simulink model "Vehicle_Model_2Track_ABS_ESP_KINOBS_EMPTY"  (R2023a)
settings: Solver=ode2  StartTime=T0  StopTime=Tf  FixedStep=Ts  EnableMultiTasking=on
model workspace (MAT data in the model file):
  aKalman = Simulink.Parameter
  aKalman.DataType = 'auto'
  aKalman.Complexity = 'real'
  aKalman.Dimensions = [0 0]
  slipEnabler = Simulink.Parameter
  slipEnabler.DataType = 'auto'
  slipEnabler.Complexity = 'real'
  slipEnabler.Dimensions = [0 0]
values from neighbouring files (symbols this model uses):
  enable_onlinePlots = 0    [run_simulation.m]
  enable_zoom = 1    [run_simulation.m]
  LLC_sampleTime = LLC.sample_time    [run_simulation.m]
  longCTRparam = longitController()    [run_simulation.m]
  previewPointParams = previewPointControllerParams()    [run_simulation.m]
  road_data_sampled = [scenario_data.path.x_sampled', scenario_data.path.y_sampled']    [run_simulation.m]
  scenario_data = load(strcat('./Scenario/', scenario_name , '.mat'))    [run_simulation.m]
  T0 = scenario_data.times.t0    [run_simulation.m]
  tau_delta = vehicle_data.steering_system.tau_D    [run_simulation.m]
  Tf = scenario_data.times.tf    [run_simulation.m]
  Ts = scenario_data.times.step_size*100    [run_simulation.m]
  vehicle_data = getVehicleDataStruct()    [run_simulation.m]
  X0 = loadInitialConditions(scenario_data.vehicle_control.max_speed/3.6)    [run_simulation.m]
undefined symbols (not defined in the file or in its folder): DiscIntNeverNeededParam, latContr_select
libraries: simulink_extras x20, simulink x9, drivingvehiclecontroller x2
(part 1 of 2)
settings Model: Creator=Edoardo  LastModifiedBy=Alessandro
settings SolverCC: AlgebraicLoopSolver=TrustRegion
settings DataIOCC: LimitDataPoints=on  SaveFormat=Array
settings OptimizationCC: DefaultParameterBehavior=Inlined  ReuseModelBlockBuffer=off  PassReuseOutputArgsAs=Individual arguments  MaxStackSize=64  EfficientTunableParamExpr=on
settings DebuggingCC: ReadBeforeWriteMsg=DisableAll  WriteAfterWriteMsg=DisableAll  WriteAfterReadMsg=DisableAll  MultiTaskDSMMsg=none  ParameterTunabilityLossMsg=error  UnconnectedInputMsg=warning  UnconnectedOutputMsg=warning  UnconnectedLineMsg=warning  PregeneratedLibrarySubsystemCodeDiagnostic=none  SFUnexpectedBacktrackingDiag=warning  SFNoUnconditionalDefaultTransitionDiag=warning  SFExecutionAtInitializationDiag=none  ArithmeticOperatorsInVariantConditions=warning
settings HardwareCC: ProdBitPerInt=16  ProdBitPerPointer=16  ProdBitPerSizeT=16  ProdBitPerPtrDiffT=16  ProdLargestAtomicFloat=None  ProdWordSize=16  ProdHWDeviceType=STMicroelectronics->ST10/Super10
settings ModelReferenceCC: UpdateModelReferenceTargets=IfOutOfDate  EnableRefExpFcnMdlSchedulingChecks=on  PropagateSignalLabelsOutOfModel=off
settings SFSimCC: SFSimEcho=off  SimUseLocalCustomCode=off  MATLABDynamicMemAlloc=off  CustomCodeUndefinedFunction=UseInterfaceOnly
settings RTWCC: Description=Embedded Coder  SystemTargetFile=ert.tlc  TemplateMakefile=ert_default_tmf  GenerateReport=on  RetainRTWFile=on  RTWUseLocalCustomCode=off  Toolchain=GNU Tools for ARM Embedded Processors  BuildConfiguration=Faster Runs  IncludeHyperlinkInReport=on  LaunchReport=on  GenerateTraceInfo=on  GenerateTraceReport=on  GenerateTraceReportSl=on  GenerateTraceReportSf=on  GenerateTraceReportEml=on  DLArmComputeVersion=19.05
settings CodeAppCC: ForceParamTrailComments=on  IgnoreCustomStorageClasses=off  OperatorAnnotations=on  SimulinkDataObjDesc=on  SFDataObjDesc=on  InsertBlockDesc=on
settings ERTTargetCC: CodeReplacementLibrary=ARM Cortex-M (Optimized)  SupportVariableSizeSignals=on  RootIOFormat=Structure reference  ERTCustomFileTemplate=example_file_process.tlc
settings ConfigComp: CovMetricSettings=dw  CovSaveCumulativeToWorkspaceVar=on  CovSaveSingleToWorkspaceVar=on  CovExternalEMLEnable=off

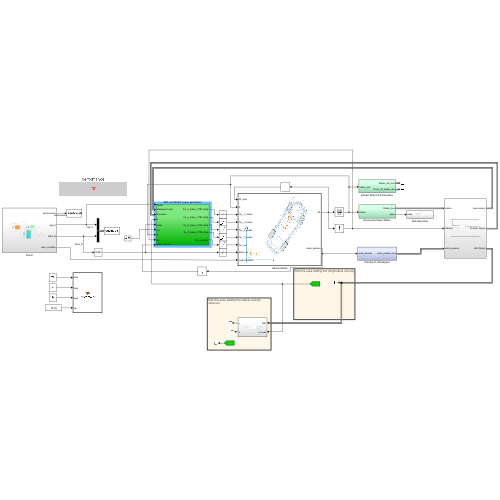
[thumbnail: Simulink's stored preview of the top-level diagram]
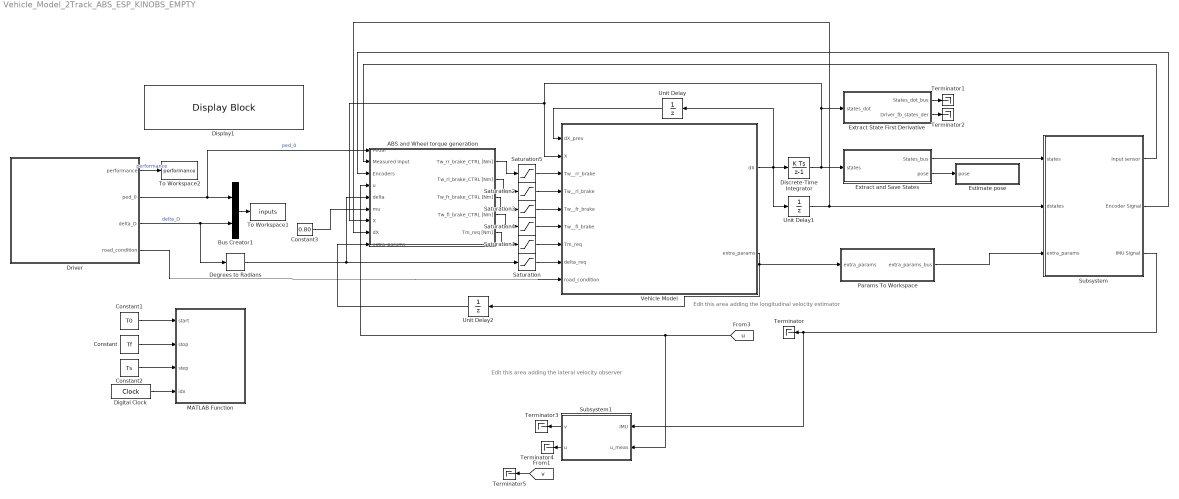
== system Vehicle_Model_2Track_ABS_ESP_KINOBS_EMPTY ==
  note: Edit this area adding the longitudinal velocity estimator
  note: Edit this area adding the lateral velocity
      | observer
  ABS and Wheel torque generation : Subsystem
  Bus Creator1 : BusCreator  Inputs=2
  Constant : Constant  Value=Tf
  Constant1 : Constant  Value=T0
  Constant2 : Constant  Value=Ts
  Constant3 : Constant  Value=0.80
  Degrees to Radians : simulink_extras/Transformations/Degrees to Radians
  Digital Clock : DigitalClock
  Discrete-Time Integrator : DiscreteIntegrator  gainval=1  InitialCondition=X0  SampleTime=-1  ICPrevOutput=DiscIntNeverNeededParam  ICPrevScaledInput=DiscIntNeverNeededParam
  Display1 : DisplayBlock  Format=Integer  Transparency=1  Layout=Fill available space
  Driver : Subsystem
  Estimate pose : Subsystem
  Extract State First Derivative : Subsystem
  Extract and Save States : Subsystem
  MATLAB Function : MATLAB Function  TreatAsAtomicUnit=on
  Params To Workspace : Subsystem
  Saturation : Saturate  UpperLimit=7  LowerLimit=-7
  Saturation1 : Saturate  UpperLimit=vehicle_data.motor.maxTorque  LowerLimit=0
  Saturation{2..5} (4 alike) : Saturate  UpperLimit=0  LowerLimit=-vehicle_data.braking.totBrakeTorque
  Subsystem : Subsystem
  Subsystem1 : Subsystem
  Terminator{,1..5} (6 alike) : Terminator
  To Workspace1 : ToWorkspace  VariableName=inputs  SaveFormat=Timeseries  SampleTime=-1
  To Workspace2 : ToWorkspace  VariableName=performance  SaveFormat=Timeseries  SampleTime=-1
  Unit Delay : UnitDelay  InitialCondition=zeros(size(X0))  SampleTime=-1  HasFrameUpgradeWarning=on
  Unit Delay1 : UnitDelay  InitialCondition=zeros(size(X0))  SampleTime=-1  HasFrameUpgradeWarning=on
  Unit Delay2 : UnitDelay  InitialCondition=zeros(size(X0))  SampleTime=-1  HasFrameUpgradeWarning=on
  Vehicle Model : MATLAB Function  TreatAsAtomicUnit=on
  wires:
  ABS and Wheel torque generation/1(Tw_rr_brake_CTRL [Nm]) -> Saturation5/1
  Subsystem/1(Input sensor) -> ABS and Wheel torque generation/2(Measured Input)
  Degrees to Radians/1 -> ABS and Wheel torque generation/5(delta), Saturation/1
  Bus Creator1/1 -> To Workspace1/1
  Extract and Save States/1(States_bus) -> Subsystem/1(states)
  ABS and Wheel torque generation/3(Tw_fr_brake_CTRL [Nm]) -> Saturation3/1
  Vehicle Model/1(dX) -> Unit Delay1/1, Unit Delay/1, Discrete-Time Integrator/1
  Extract State First Derivative/2(Driver_fb_states_der) -> Terminator2/1
  Subsystem/2(Encoder Signal) -> ABS and Wheel torque generation/3(Encoders)
  Unit Delay/1 -> Vehicle Model/1(dX_prev)
  Extract State First Derivative/1(States_dot_bus) -> Terminator1/1
  Driver/3(delta_D) -> Degrees to Radians/1, Bus Creator1/2  "delta_D"
  Vehicle Model/2(extra_params) -> Unit Delay2/1, Params To Workspace/1(extra_params)
  ABS and Wheel torque generation/2(Tw_rl_brake_CTRL [Nm]) -> Saturation2/1
  ABS and Wheel torque generation/5(Tm_req [Nm]) -> Saturation1/1
  Driver/2(ped_0) -> ABS and Wheel torque generation/1(Pedal), Bus Creator1/1  "ped_0"
  ABS and Wheel torque generation/4(Tw_fl_brake_CTRL [Nm]) -> Saturation4/1
  Params To Workspace/1(extra_params_bus) -> Subsystem/3(extra_params)
  Constant/1 -> MATLAB Function/2(stop)
  Constant1/1 -> MATLAB Function/1(start)
  Digital Clock/1 -> MATLAB Function/4(idx)
  Constant2/1 -> MATLAB Function/3(step)
  Extract and Save States/2(pose) -> Estimate pose/1(pose)
  [u] -> Subsystem1/2(u_meas), ABS and Wheel torque generation/4(u)
  Saturation/1 -> Vehicle Model/8(delta_req)
  Driver/4(road_condition) -> Vehicle Model/9(road_condition)
  Subsystem/3(IMU Signal) -> Subsystem1/1(IMU), Terminator/1
  Saturation1/1 -> Vehicle Model/7(Tm_req)
  Saturation4/1 -> Vehicle Model/6(Tw__fl_brake)
  Saturation3/1 -> Vehicle Model/5(Tw__fr_brake)
  Saturation2/1 -> Vehicle Model/4(Tw__rl_brake)
  Saturation5/1 -> Vehicle Model/3(Tw__rr_brake)
  Driver/1(performance) -> To Workspace2/1  "performance"
  Unit Delay1/1 -> ABS and Wheel torque generation/8(dX), Subsystem/2(dstates)
  [v] -> Terminator5/1
  Constant3/1 -> ABS and Wheel torque generation/6(mu)
  Subsystem1/1(v) -> Terminator3/1
  Subsystem1/2(u) -> Terminator4/1
  Unit Delay2/1 -> ABS and Wheel torque generation/9(extra_params)
  Discrete-Time Integrator/1 -> Extract and Save States/1(states), Extract State First Derivative/1(states_dot), ABS and Wheel torque generation/7(X), Vehicle Model/2(X)

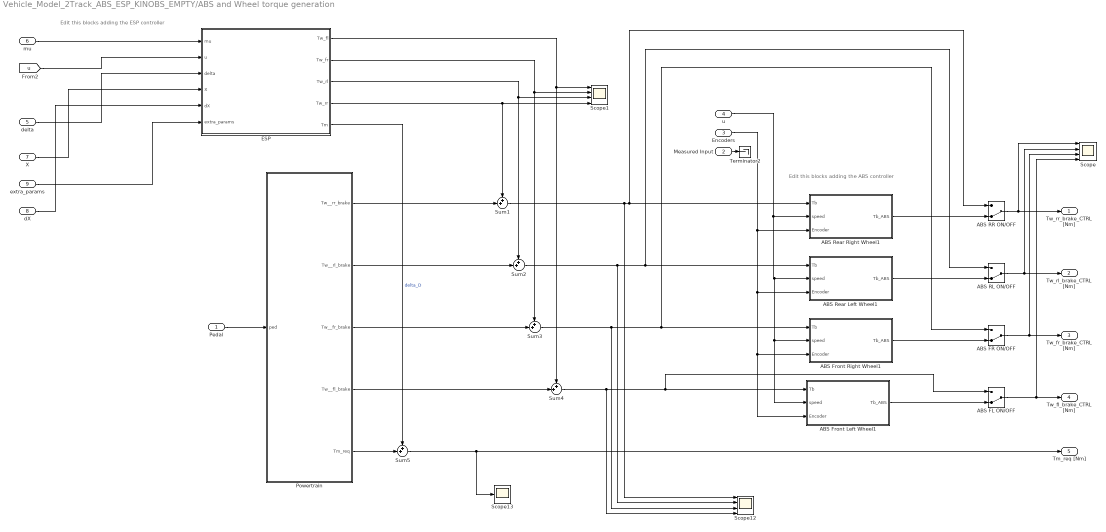
== system Vehicle_Model_2Track_ABS_ESP_KINOBS_EMPTY/ABS and Wheel torque generation ==
  note: Edit this blocks adding the ESP controller
  note: Edit this blocks adding the ABS controller
  Pedal : Inport
  Measured Input : Inport  Port=2
  Encoders : Inport  Port=3
  u : Inport  Port=4
  delta : Inport  Port=5
  mu : Inport  Port=6
  X : Inport  Port=7
  dX : Inport  Port=8
  extra_params : Inport  Port=9
  ABS FL ON/OFF : ManualSwitch  CurrentSetting=0
  ABS FR ON/OFF : ManualSwitch  CurrentSetting=0
  ABS Front Left Wheel1 : Subsystem
  ABS Front Right Wheel1 : Subsystem
  ABS RL ON/OFF : ManualSwitch  CurrentSetting=0
  ABS RR ON/OFF : ManualSwitch  CurrentSetting=0
  ABS Rear Left Wheel1 : Subsystem
  ABS Rear Right Wheel1 : Subsystem
  ESP : Subsystem
  Powertrain : MATLAB Function  TreatAsAtomicUnit=on
  Scope : Scope  NumInputPorts=4
  Scope1 : Scope  NumInputPorts=4
  Scope12 : Scope  NumInputPorts=4
  Scope13 : Scope
  Sum{1..5} (5 alike) : Sum  Inputs=++|
  Terminator2 : Terminator
  Tw_rr_brake_CTRL [Nm] : Outport  VectorParamsAs1DForOutWhenUnconnected=off
  Tw_rl_brake_CTRL [Nm] : Outport  Port=2  VectorParamsAs1DForOutWhenUnconnected=off
  Tw_fr_brake_CTRL [Nm] : Outport  Port=3  VectorParamsAs1DForOutWhenUnconnected=off
  Tw_fl_brake_CTRL [Nm] : Outport  Port=4  VectorParamsAs1DForOutWhenUnconnected=off
  Tm_req [Nm] : Outport  Port=5  VectorParamsAs1DForOutWhenUnconnected=off
  wires:
  Sum3/1 -> Scope12/3, ABS Front Right Wheel1/1(Tb), ABS FR ON/OFF/1
  ABS FL ON/OFF/1 -> Tw_fl_brake_CTRL [Nm]/1, Scope/4
  Sum5/1 -> Scope13/1, Tm_req [Nm]/1
  ABS FR ON/OFF/1 -> Tw_fr_brake_CTRL [Nm]/1, Scope/3
  u/1 -> ABS Rear Right Wheel1/2(speed), ABS Rear Left Wheel1/2(speed), ABS Front Right Wheel1/2(speed), ABS Front Left Wheel1/2(speed)
  ABS RL ON/OFF/1 -> Tw_rl_brake_CTRL [Nm]/1, Scope/2
  Sum2/1 -> Scope12/2, ABS Rear Left Wheel1/1(Tb), ABS RL ON/OFF/1
  Pedal/1 -> Powertrain/1(ped)
  ABS RR ON/OFF/1 -> Scope/1, Tw_rr_brake_CTRL [Nm]/1
  Encoders/1 -> ABS Rear Right Wheel1/3(Encoder), ABS Rear Left Wheel1/3(Encoder), ABS Front Right Wheel1/3(Encoder), ABS Front Left Wheel1/3(Encoder)
  Measured Input/1 -> Terminator2/1
  Sum4/1 -> ABS FL ON/OFF/1, ABS Front Left Wheel1/1(Tb), Scope12/4
  ABS Front Left Wheel1/1(Tb_ABS) -> ABS FL ON/OFF/2
  Sum1/1 -> Scope12/1, ABS Rear Right Wheel1/1(Tb), ABS RR ON/OFF/1
  Powertrain/1(Tw__rr_brake) -> Sum1/2
  Powertrain/2(Tw__rl_brake) -> Sum2/2
  Powertrain/3(Tw__fr_brake) -> Sum3/2
  Powertrain/4(Tw__fl_brake) -> Sum4/2
  Powertrain/5(Tm_req) -> Sum5/2
  ESP/5(Tm) -> Sum5/1  "delta_D"
  ESP/1(Tw_fl) -> Sum4/1, Scope1/1
  ESP/3(Tw_rl) -> Sum2/1, Scope1/3
  ESP/2(Tw_fr) -> Sum3/1, Scope1/2
  ESP/4(Tw_rr) -> Sum1/1, Scope1/4
  mu/1 -> ESP/1(mu)
  [u] -> ESP/2(u)
  delta/1 -> ESP/3(delta)
  ABS Front Right Wheel1/1(Tb_ABS) -> ABS FR ON/OFF/2
  ABS Rear Left Wheel1/1(Tb_ABS) -> ABS RL ON/OFF/2
  ABS Rear Right Wheel1/1(Tb_ABS) -> ABS RR ON/OFF/2
  X/1 -> ESP/4(X)
  dX/1 -> ESP/5(dX)
  extra_params/1 -> ESP/6(extra_params)

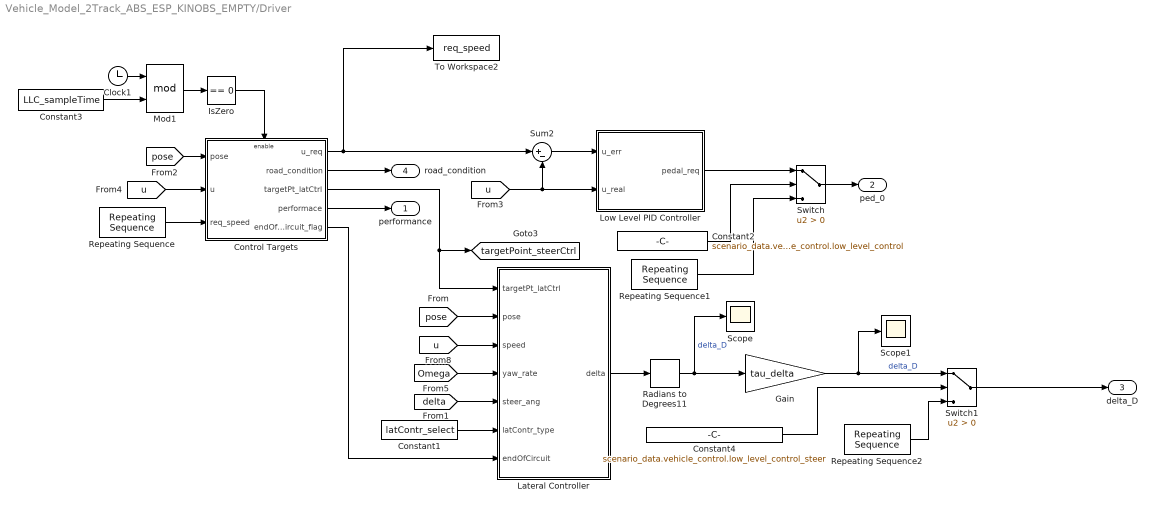
== system Vehicle_Model_2Track_ABS_ESP_KINOBS_EMPTY/Driver ==
  Clock1 : Clock
  Constant1 : Constant  Value=latContr_select
  Constant2 : Constant  Value=scenario_data.vehicle_control.low_level_control
  Constant3 : Constant  Value=LLC_sampleTime
  Constant4 : Constant  Value=scenario_data.vehicle_control.low_level_control_steer
  Control Targets : Subsystem
  Gain : Gain  Gain=tau_delta
  IsZero : simulink/Logic and Bit Operations/Compare To Zero  relop===  OutDataTypeStr=boolean
  Lateral Controller : Subsystem
  Low Level PID Controller : Subsystem
  Mod1 : Math  Operator=mod  SignedPower=on
  Radians to Degrees11 : simulink_extras/Transformations/Radians to Degrees
  Repeating Sequence : simulink/Sources/Repeating Sequence  rep_seq_t=scenario_data.vehicle_control.time_manoeuvre  rep_seq_y=scenario_data.vehicle_control.req_speed
  Repeating Sequence1 : simulink/Sources/Repeating Sequence  rep_seq_t=scenario_data.vehicle_control.time_pedal  rep_seq_y=scenario_data.vehicle_control.req_pedal
  Repeating Sequence2 : simulink/Sources/Repeating Sequence  rep_seq_t=scenario_data.vehicle_control.time_delta  rep_seq_y=scenario_data.vehicle_control.req_delta
  Scope : Scope
  Scope1 : Scope
  Sum2 : Sum  Inputs=|+-
  Switch : Switch  Criteria=u2 > Threshold  SaturateOnIntegerOverflow=off  InputSameDT=off
  Switch1 : Switch  Criteria=u2 > Threshold  SaturateOnIntegerOverflow=off  InputSameDT=off
  To Workspace2 : ToWorkspace  VariableName=req_speed  SaveFormat=Timeseries  SampleTime=-1
  performance : Outport
  ped_0 : Outport  Port=2  PortDimensions=1
  delta_D : Outport  Port=3  PortDimensions=1
  road_condition : Outport  Port=4
  tag scope: targetPoint_steerCtrl=global
  wires:
  Constant1/1 -> Lateral Controller/6(latContr_type)
  [pose] -> Lateral Controller/2(pose)
  [pose] -> Control Targets/1(pose)
  IsZero/1 -> Control Targets/Enable
  [u] -> Lateral Controller/3(speed)
  [u] -> Sum2/2, Low Level PID Controller/2(u_real)
  Clock1/1 -> Mod1/1
  Control Targets/1(u_req) -> Sum2/1, To Workspace2/1
  [Omega] -> Lateral Controller/4(yaw_rate)
  Sum2/1 -> Low Level PID Controller/1(u_err)
  Constant3/1 -> Mod1/2
  Mod1/1 -> IsZero/1
  Control Targets/3(targetPt_latCtrl) -> Lateral Controller/1(targetPt_latCtrl), [targetPoint_steerCtrl]
  [delta] -> Lateral Controller/5(steer_ang)
  Lateral Controller/1(delta) -> Radians to Degrees11/1
  Control Targets/5(endOfCircuit_flag) -> Lateral Controller/7(endOfCircuit)
  Gain/1 -> Switch1/1, Scope1/1  "delta_D"
  Repeating Sequence/1 -> Control Targets/3(req_speed)
  Switch/1 -> ped_0/1
  Repeating Sequence1/1 -> Switch/3
  Low Level PID Controller/1(pedal_req) -> Switch/1
  Radians to Degrees11/1 -> Gain/1, Scope/1  "delta_D"
  Control Targets/2(road_condition) -> road_condition/1
  Constant2/1 -> Switch/2
  Constant4/1 -> Switch1/2
  Repeating Sequence2/1 -> Switch1/3
  Switch1/1 -> delta_D/1
  [u] -> Control Targets/2(u)
  Control Targets/4(performace) -> performance/1

== system Vehicle_Model_2Track_ABS_ESP_KINOBS_EMPTY/Estimate pose ==
  pose : Inport
  Constant3 : Constant  Value=enable_onlinePlots
  Online Trajectory Plots : Subsystem
      mask Display: image('example_path.png'); % Use "Edit Image" on toolstrip to change.
  To Workspace4 : ToWorkspace  VariableName=vehicle_pose  SampleTime=-1
      settings: Save2DSignal=2-D array (concatenate along first dimension)
  wires:
  [targetPoint_steerCtrl] -> Online Trajectory Plots/1(targetPoint_steerCtrl)
  Constant3/1 -> Online Trajectory Plots/Enable
  pose/1 -> To Workspace4/1, Online Trajectory Plots/2(pose)

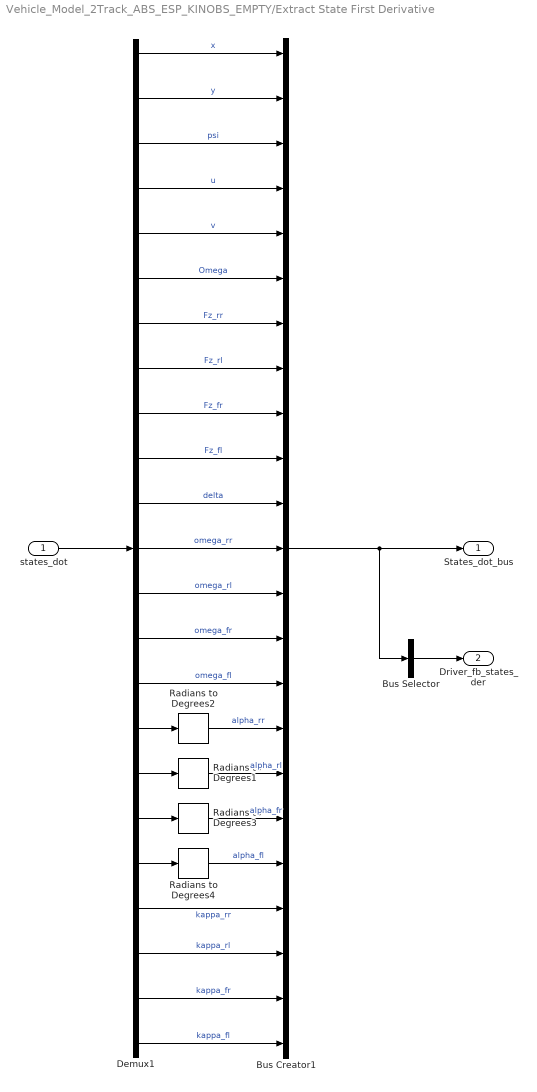
== system Vehicle_Model_2Track_ABS_ESP_KINOBS_EMPTY/Extract State First Derivative ==
  states_dot : Inport
  Bus Creator1 : BusCreator  Inputs=23
  Bus Selector : BusSelector  OutputSignals=Omega,x,y,u  OutputAsBus=on
  Demux1 : Demux  Outputs=23
  Radians to Degrees{1..4} (4 alike) : simulink_extras/Transformations/Radians to Degrees
  States_dot_bus : Outport
  Driver_fb_states_der : Outport  Port=2
  wires:
  Demux1/13 -> Bus Creator1/13  "omega_rl"
  Demux1/8 -> Bus Creator1/8  "Fz_rl"
  Demux1/23 -> Bus Creator1/23  "kappa_fl"
  Demux1/19 -> Radians to Degrees4/1
  states_dot/1 -> Demux1/1
  Demux1/14 -> Bus Creator1/14  "omega_fr"
  Demux1/7 -> Bus Creator1/7  "Fz_rr"
  Demux1/15 -> Bus Creator1/15  "omega_fl"
  Demux1/3 -> Bus Creator1/3  "psi"
  Demux1/22 -> Bus Creator1/22  "kappa_fr"
  Demux1/4 -> Bus Creator1/4  "u"
  Demux1/6 -> Bus Creator1/6  "Omega"
  Demux1/11 -> Bus Creator1/11  "delta"
  Demux1/5 -> Bus Creator1/5  "v"
  Demux1/9 -> Bus Creator1/9  "Fz_fr"
  Demux1/21 -> Bus Creator1/21  "kappa_rl"
  Demux1/12 -> Bus Creator1/12  "omega_rr"
  Demux1/17 -> Radians to Degrees1/1
  Demux1/2 -> Bus Creator1/2  "y"
  Demux1/20 -> Bus Creator1/20  "kappa_rr"
  Demux1/10 -> Bus Creator1/10  "Fz_fl"
  Demux1/18 -> Radians to Degrees3/1
  Demux1/1 -> Bus Creator1/1  "x"
  Demux1/16 -> Radians to Degrees2/1
  Bus Creator1/1 -> Bus Selector/1, States_dot_bus/1
  Radians to Degrees2/1 -> Bus Creator1/16  "alpha_rr"
  Radians to Degrees1/1 -> Bus Creator1/17  "alpha_rl"
  Radians to Degrees3/1 -> Bus Creator1/18  "alpha_fr"
  Radians to Degrees4/1 -> Bus Creator1/19  "alpha_fl"
  Bus Selector/1 -> Driver_fb_states_der/1

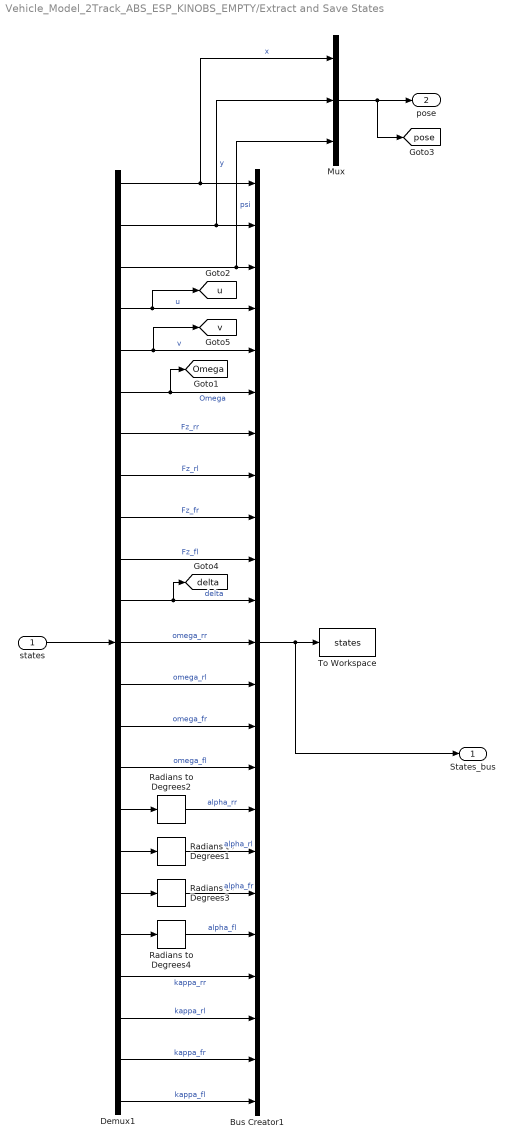
== system Vehicle_Model_2Track_ABS_ESP_KINOBS_EMPTY/Extract and Save States ==
  states : Inport
  Bus Creator1 : BusCreator  Inputs=23
  Demux1 : Demux  Outputs=23
  Mux : Mux  Inputs=3
  Radians to Degrees{1..4} (4 alike) : simulink_extras/Transformations/Radians to Degrees
  To Workspace : ToWorkspace  VariableName=states  SaveFormat=Timeseries  SampleTime=-1
  States_bus : Outport
  pose : Outport  Port=2
  tag scope: Omega=global, delta=global, pose=global, u=global, v=global
  wires:
  Demux1/13 -> Bus Creator1/13  "omega_rl"
  Demux1/8 -> Bus Creator1/8  "Fz_rl"
  Demux1/23 -> Bus Creator1/23  "kappa_fl"
  Demux1/19 -> Radians to Degrees4/1
  states/1 -> Demux1/1
  Demux1/14 -> Bus Creator1/14  "omega_fr"
  Demux1/7 -> Bus Creator1/7  "Fz_rr"
  Demux1/15 -> Bus Creator1/15  "omega_fl"
  Demux1/22 -> Bus Creator1/22  "kappa_fr"
  Demux1/6 -> [Omega], Bus Creator1/6  "Omega"
  Demux1/11 -> [delta], Bus Creator1/11  "delta"
  Demux1/5 -> [v], Bus Creator1/5  "v"
  Demux1/9 -> Bus Creator1/9  "Fz_fr"
  Demux1/21 -> Bus Creator1/21  "kappa_rl"
  Demux1/12 -> Bus Creator1/12  "omega_rr"
  Demux1/17 -> Radians to Degrees1/1
  Demux1/20 -> Bus Creator1/20  "kappa_rr"
  Demux1/10 -> Bus Creator1/10  "Fz_fl"
  Demux1/18 -> Radians to Degrees3/1
  Demux1/16 -> Radians to Degrees2/1
  Bus Creator1/1 -> States_bus/1, To Workspace/1
  Radians to Degrees2/1 -> Bus Creator1/16  "alpha_rr"
  Radians to Degrees1/1 -> Bus Creator1/17  "alpha_rl"
  Radians to Degrees3/1 -> Bus Creator1/18  "alpha_fr"
  Radians to Degrees4/1 -> Bus Creator1/19  "alpha_fl"
  Demux1/1 -> Mux/1, Bus Creator1/1  "x"
  Demux1/3 -> Mux/3, Bus Creator1/3  "psi"
  Demux1/4 -> [u], Bus Creator1/4  "u"
  Demux1/2 -> Bus Creator1/2, Mux/2  "y"
  Mux/1 -> [pose], pose/1

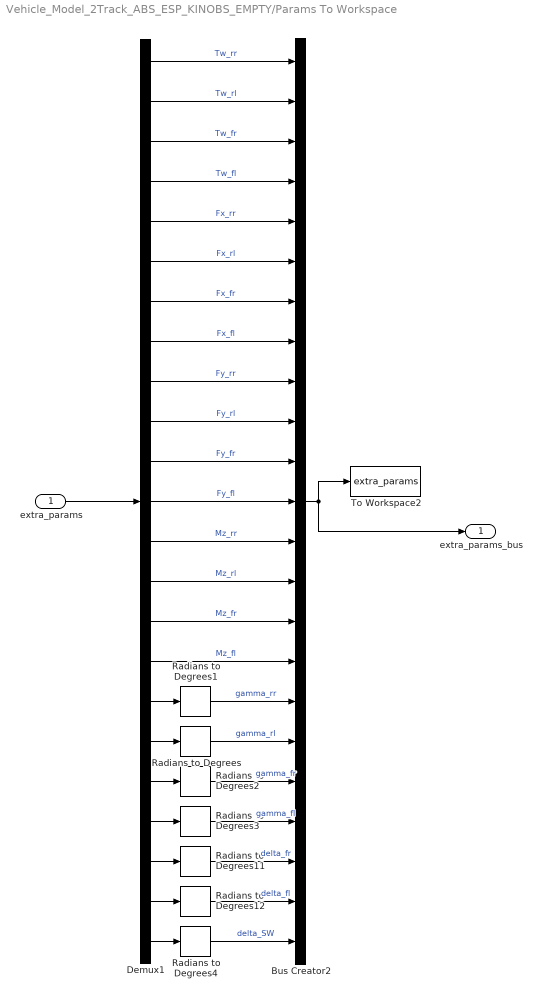
== system Vehicle_Model_2Track_ABS_ESP_KINOBS_EMPTY/Params To Workspace ==
  extra_params : Inport
  Bus Creator2 : BusCreator  Inputs=23
  Demux1 : Demux  Outputs=23
  Radians to Degrees{,1..4,11..12} (7 alike) : simulink_extras/Transformations/Radians to Degrees
  To Workspace2 : ToWorkspace  VariableName=extra_params  SaveFormat=Timeseries  SampleTime=-1
  extra_params_bus : Outport
  wires:
  Demux1/17 -> Radians to Degrees1/1
  Demux1/3 -> Bus Creator2/3  "Tw_fr"
  Radians to Degrees3/1 -> Bus Creator2/20  "gamma_fl"
  Demux1/16 -> Bus Creator2/16  "Mz_fl"
  Radians to Degrees1/1 -> Bus Creator2/17  "gamma_rr"
  Radians to Degrees11/1 -> Bus Creator2/21  "delta_fr"
  Demux1/14 -> Bus Creator2/14  "Mz_rl"
  Demux1/4 -> Bus Creator2/4  "Tw_fl"
  Demux1/6 -> Bus Creator2/6  "Fx_rl"
  Demux1/8 -> Bus Creator2/8  "Fx_fl"
  Demux1/13 -> Bus Creator2/13  "Mz_rr"
  Demux1/7 -> Bus Creator2/7  "Fx_fr"
  Demux1/5 -> Bus Creator2/5  "Fx_rr"
  Demux1/9 -> Bus Creator2/9  "Fy_rr"
  Demux1/11 -> Bus Creator2/11  "Fy_fr"
  Demux1/15 -> Bus Creator2/15  "Mz_fr"
  Demux1/10 -> Bus Creator2/10  "Fy_rl"
  Radians to Degrees12/1 -> Bus Creator2/22  "delta_fl"
  Radians to Degrees2/1 -> Bus Creator2/19  "gamma_fr"
  extra_params/1 -> Demux1/1
  Demux1/12 -> Bus Creator2/12  "Fy_fl"
  Bus Creator2/1 -> To Workspace2/1, extra_params_bus/1
  Demux1/1 -> Bus Creator2/1  "Tw_rr"
  Demux1/2 -> Bus Creator2/2  "Tw_rl"
  Radians to Degrees/1 -> Bus Creator2/18  "gamma_rl"
  Demux1/18 -> Radians to Degrees/1
  Demux1/19 -> Radians to Degrees2/1
  Demux1/20 -> Radians to Degrees3/1
  Demux1/21 -> Radians to Degrees11/1
  Demux1/22 -> Radians to Degrees12/1
  Demux1/23 -> Radians to Degrees4/1
  Radians to Degrees4/1 -> Bus Creator2/23  "delta_SW"

== system Vehicle_Model_2Track_ABS_ESP_KINOBS_EMPTY/Subsystem ==
  states : Inport
  dstates : Inport  Port=2
  extra_params : Inport  Port=3
  Bus Selector : BusSelector  OutputSignals=omega_rr,omega_rl,omega_fr,omega_fl  OutputAsBus=on
  Bus Selector1 : BusSelector  OutputSignals=delta_SW,Tw_rr,Tw_rl,Tw_fr,Tw_fl  OutputAsBus=on
  IMU1 : Subsystem
  Input sensor : Outport  VectorParamsAs1DForOutWhenUnconnected=off
  Encoder Signal : Outport  Port=2  VectorParamsAs1DForOutWhenUnconnected=off
  IMU Signal : Outport  Port=3  VectorParamsAs1DForOutWhenUnconnected=off
  wires:
  states/1 -> IMU1/1(states), Bus Selector/1
  Bus Selector/1 -> Encoder Signal/1
  IMU1/1(IMU) -> IMU Signal/1
  extra_params/1 -> Bus Selector1/1
  Bus Selector1/1 -> Input sensor/1
  dstates/1 -> IMU1/2(dstates)

== system Vehicle_Model_2Track_ABS_ESP_KINOBS_EMPTY/Subsystem1 ==
  IMU : Inport
  u_meas : Inport  Port=2
  Bus Selector : BusSelector  OutputSignals=a_x,a_y,Omega
  Demux : Demux  Outputs=2
  Discrete-Time Integrator : DiscreteIntegrator  InitialCondition=[0 ; 0]  SampleTime=-1  ICPrevOutput=DiscIntNeverNeededParam  ICPrevScaledInput=DiscIntNeverNeededParam
  MATLAB Function : MATLAB Function  TreatAsAtomicUnit=on
  gamma : Constant
  v : Outport
  u : Outport  Port=2
  wires:
  IMU/1 -> Bus Selector/1
  Bus Selector/3 -> MATLAB Function/4(omega)  "<Omega>"
  Bus Selector/2 -> MATLAB Function/3(ay)  "<a_y>"
  Bus Selector/1 -> MATLAB Function/2(ax)  "<a_x>"
  MATLAB Function/1(X_dot) -> Discrete-Time Integrator/1
  Discrete-Time Integrator/1 -> MATLAB Function/1(X), Demux/1
  Demux/1 -> v/1
  Demux/2 -> u/1
  gamma/1 -> MATLAB Function/5(gamma)
  u_meas/1 -> MATLAB Function/6(u_meas)

== system Vehicle_Model_2Track_ABS_ESP_KINOBS_EMPTY/ABS and Wheel torque generation/ABS Front Left Wheel1 ==
  Tb : Inport
  speed : Inport  Port=2
  Encoder : Inport  Port=3
  Terminator : Terminator
  Terminator1 : Terminator
  To Workspace3 : ToWorkspace  VariableName=TwrflCtrl  SaveFormat=Timeseries  SampleTime=-1
  Tb_ABS : Outport  VectorParamsAs1DForOutWhenUnconnected=off
  wires:
  Encoder/1 -> Terminator/1
  Tb/1 -> To Workspace3/1, Tb_ABS/1
  speed/1 -> Terminator1/1

== system Vehicle_Model_2Track_ABS_ESP_KINOBS_EMPTY/ABS and Wheel torque generation/ABS Front Right Wheel1 ==
  Tb : Inport
  speed : Inport  Port=2
  Encoder : Inport  Port=3
  Terminator : Terminator
  Terminator1 : Terminator
  To Workspace3 : ToWorkspace  VariableName=TwfrCtrl  SaveFormat=Timeseries  SampleTime=-1
  Tb_ABS : Outport  VectorParamsAs1DForOutWhenUnconnected=off
  wires:
  Encoder/1 -> Terminator1/1
  Tb/1 -> Tb_ABS/1, To Workspace3/1
  speed/1 -> Terminator/1

== system Vehicle_Model_2Track_ABS_ESP_KINOBS_EMPTY/ABS and Wheel torque generation/ABS Rear Left Wheel1 ==
  Tb : Inport
  speed : Inport  Port=2
  Encoder : Inport  Port=3
  Terminator : Terminator
  Terminator1 : Terminator
  To Workspace3 : ToWorkspace  VariableName=TwrlCtrl  SaveFormat=Timeseries  SampleTime=-1
  Tb_ABS : Outport  VectorParamsAs1DForOutWhenUnconnected=off
  wires:
  Encoder/1 -> Terminator1/1
  Tb/1 -> To Workspace3/1, Tb_ABS/1
  speed/1 -> Terminator/1

== system Vehicle_Model_2Track_ABS_ESP_KINOBS_EMPTY/ABS and Wheel torque generation/ABS Rear Right Wheel1 ==
  Tb : Inport
  speed : Inport  Port=2
  Encoder : Inport  Port=3
  Terminator : Terminator
  Terminator1 : Terminator
  To Workspace3 : ToWorkspace  VariableName=TwrrCtrl  SaveFormat=Timeseries  SampleTime=-1
  Tb_ABS : Outport  VectorParamsAs1DForOutWhenUnconnected=off
  wires:
  Encoder/1 -> Terminator1/1
  Tb/1 -> To Workspace3/1, Tb_ABS/1
  speed/1 -> Terminator/1

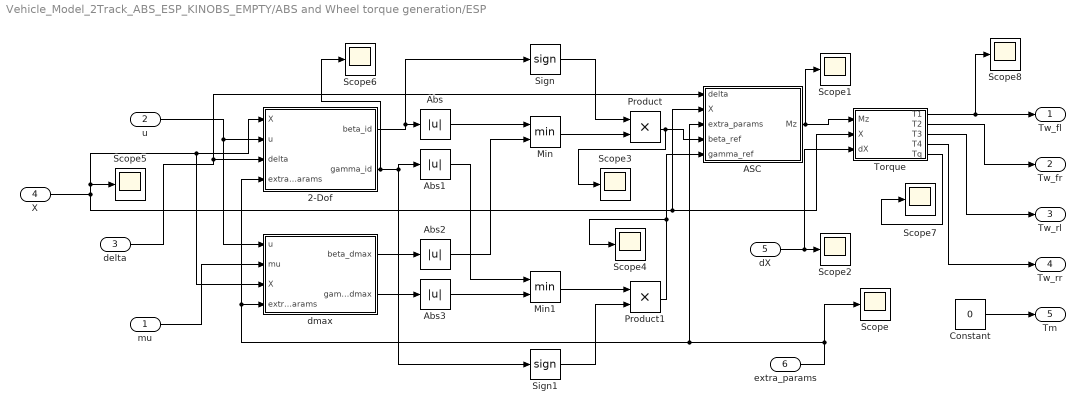
== system Vehicle_Model_2Track_ABS_ESP_KINOBS_EMPTY/ABS and Wheel torque generation/ESP ==
  mu : Inport
  u : Inport  Port=2
  delta : Inport  Port=3
  X : Inport  Port=4
  dX : Inport  Port=5
  extra_params : Inport  Port=6
  2-Dof : MATLAB Function  TreatAsAtomicUnit=on
  ASC : MATLAB Function  TreatAsAtomicUnit=on
  Abs{,1..3} (4 alike) : Abs  SaturateOnIntegerOverflow=off
  Constant : Constant  Value=0
  Min : MinMax  Inputs=2
  Min1 : MinMax  Inputs=2
  Product : Product
  Product1 : Product
  Scope{,1..8} (9 alike) : Scope
  Sign : Signum
  Sign1 : Signum
  Torque : MATLAB Function  TreatAsAtomicUnit=on
  dmax : MATLAB Function  TreatAsAtomicUnit=on
  Tw_fl : Outport
  Tw_fr : Outport  Port=2
  Tw_rl : Outport  Port=3
  Tw_rr : Outport  Port=4
  Tm : Outport  Port=5
  wires:
  mu/1 -> dmax/2(mu)
  dmax/1(beta_dmax) -> Abs2/1
  dmax/2(gamma_dmax) -> Abs3/1
  Abs/1 -> Min/1
  Abs2/1 -> Min/2
  Abs1/1 -> Min1/1
  Abs3/1 -> Min1/2
  Sign/1 -> Product/1
  Min/1 -> Product/2
  Min1/1 -> Product1/1
  Sign1/1 -> Product1/2
  X/1 -> Torque/2(X), ASC/2(X), 2-Dof/1(X), dmax/3(X), Scope5/1
  ASC/1(Mz) -> Scope1/1, Torque/1(Mz)
  dX/1 -> Scope2/1, Torque/3(dX)
  Product/1 -> Scope3/1, ASC/4(beta_ref)
  Product1/1 -> Scope4/1, ASC/5(gamma_ref)
  Constant/1 -> Tm/1
  extra_params/1 -> Scope/1, ASC/3(extra_params), 2-Dof/4(extra_params), dmax/4(extra_params)
  2-Dof/1(beta_id) -> Sign/1, Abs/1
  2-Dof/2(gamma_id) -> Scope6/1, Abs1/1, Sign1/1
  u/1 -> 2-Dof/2(u), dmax/1(u)
  Torque/4(T4) -> Tw_rr/1
  Torque/1(T1) -> Scope8/1, Tw_fl/1
  Torque/3(T3) -> Tw_rl/1
  Torque/2(T2) -> Tw_fr/1
  delta/1 -> 2-Dof/3(delta), ASC/1(delta)
  Torque/5(Tq) -> Scope7/1

== system Vehicle_Model_2Track_ABS_ESP_KINOBS_EMPTY/Driver/Control Targets ==
  pose : Inport
  u : Inport  Port=2
  req_speed : Inport  Port=3
  Enable : EnablePort
  MATLAB System : MATLABSystem  System=setControlTargets  lateralController_type=latContr_select  purePursuit_lookAhead=purePursuitParams.lookAhead  clothoidBased_lookAhead=clothoidBasedParams.lookAhead  previewPoint_lookAhead=previewPointParams.lookAhead  refRoute_points=road_data  road_condition=road_condition  Lf=vehicle_data.vehicle.Lf  SimulateUsing=Interpreted execution
      mask Type: setControlTargets
      mask Display:
      | disp('setControlTargets');
      | port_label('input',1,'vehPose');
      | port_label('input',2,'u');
      | port_label('input',3,'req_speed');
      | port_label('output',1,'targetPoint_latControl');
      | port_label('output',2,'speed_req');
      | port_label('output',3,'road_condition');
      | port_label('output',4,'performance');
      | port_label('output',5,'endOfCircuit');
  u_req : Outport  VectorParamsAs1DForOutWhenUnconnected=off
  road_condition : Outport  Port=2
  targetPt_latCtrl : Outport  Port=3  VectorParamsAs1DForOutWhenUnconnected=off
  performace : Outport  Port=4  VectorParamsAs1DForOutWhenUnconnected=off
  endOfCircuit_flag : Outport  Port=5  VectorParamsAs1DForOutWhenUnconnected=off
  wires:
  pose/1 -> MATLAB System/1
  MATLAB System/2 -> u_req/1
  MATLAB System/1 -> targetPt_latCtrl/1
  MATLAB System/4 -> performace/1
  req_speed/1 -> MATLAB System/3
  MATLAB System/3 -> road_condition/1
  u/1 -> MATLAB System/2
  MATLAB System/5 -> endOfCircuit_flag/1

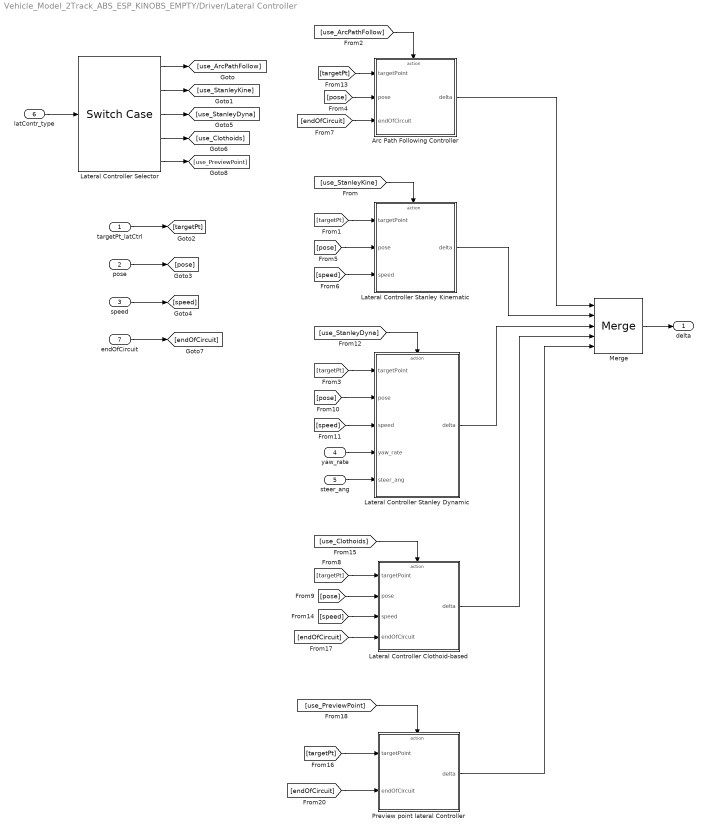
== system Vehicle_Model_2Track_ABS_ESP_KINOBS_EMPTY/Driver/Lateral Controller ==
  targetPt_latCtrl : Inport
  pose : Inport  Port=2
  speed : Inport  Port=3
  yaw_rate : Inport  Port=4
  steer_ang : Inport  Port=5
  latContr_type : Inport  Port=6
  endOfCircuit : Inport  Port=7
  Arc Path Following Controller : Subsystem  TreatAsAtomicUnit=on
  Lateral Controller Clothoid-based : Subsystem  TreatAsAtomicUnit=on
  Lateral Controller Selector : SwitchCase  CaseConditions={1,2,3,4,5}  ShowDefaultCase=off
  Lateral Controller Stanley Dynamic : Subsystem  TreatAsAtomicUnit=on
  Lateral Controller Stanley Kinematic : Subsystem  TreatAsAtomicUnit=on
  Merge : Merge  Inputs=5
  Preview point lateral Controller : Subsystem  TreatAsAtomicUnit=on
  delta : Outport  VectorParamsAs1DForOutWhenUnconnected=off
  wires:
  Arc Path Following Controller/1(delta) -> Merge/1
  latContr_type/1 -> Lateral Controller Selector/1
  Lateral Controller Stanley Kinematic/1(delta) -> Merge/2
  Merge/1 -> delta/1
  Lateral Controller Selector/1 -> [use_ArcPathFollow]
  [use_ArcPathFollow] -> Arc Path Following Controller/Action
  Lateral Controller Selector/2 -> [use_StanleyKine]
  [use_StanleyKine] -> Lateral Controller Stanley Kinematic/Action
  targetPt_latCtrl/1 -> [targetPt]
  [targetPt] -> Arc Path Following Controller/1(targetPoint)
  [targetPt] -> Lateral Controller Stanley Kinematic/1(targetPoint)
  pose/1 -> [pose]
  [pose] -> Arc Path Following Controller/2(pose)
  [pose] -> Lateral Controller Stanley Kinematic/2(pose)
  speed/1 -> [speed]
  [speed] -> Lateral Controller Stanley Kinematic/3(speed)
  Lateral Controller Selector/3 -> [use_StanleyDyna]
  [pose] -> Lateral Controller Stanley Dynamic/2(pose)
  [targetPt] -> Lateral Controller Stanley Dynamic/1(targetPoint)
  [speed] -> Lateral Controller Stanley Dynamic/3(speed)
  [use_StanleyDyna] -> Lateral Controller Stanley Dynamic/Action
  Lateral Controller Stanley Dynamic/1(delta) -> Merge/3
  yaw_rate/1 -> Lateral Controller Stanley Dynamic/4(yaw_rate)
  steer_ang/1 -> Lateral Controller Stanley Dynamic/5(steer_ang)
  [use_Clothoids] -> Lateral Controller Clothoid-based/Action
  [pose] -> Lateral Controller Clothoid-based/2(pose)
  [targetPt] -> Lateral Controller Clothoid-based/1(targetPoint)
  [speed] -> Lateral Controller Clothoid-based/3(speed)
  Lateral Controller Clothoid-based/1(delta) -> Merge/4
  Lateral Controller Selector/4 -> [use_Clothoids]
  [endOfCircuit] -> Arc Path Following Controller/3(endOfCircuit)
  [endOfCircuit] -> Lateral Controller Clothoid-based/4(endOfCircuit)
  endOfCircuit/1 -> [endOfCircuit]
  [targetPt] -> Preview point lateral Controller/1(targetPoint)
  [endOfCircuit] -> Preview point lateral Controller/2(endOfCircuit)
  [use_PreviewPoint] -> Preview point lateral Controller/Action
  Lateral Controller Selector/5 -> [use_PreviewPoint]
  Preview point lateral Controller/1(delta) -> Merge/5

== system Vehicle_Model_2Track_ABS_ESP_KINOBS_EMPTY/Driver/Low Level PID Controller ==
  u_err : Inport
  u_real : Inport  Port=2
  1-D Lookup Table : Lookup_n-D  NumberOfTableDimensions=1  BreakpointsForDimension1=longCTRparam.speed_vals_PID_sched  BeginIndexSearchUsingPreviousIndexResult=on  Table=longCTRparam.Kp_vals  ExtrapMethod=Clip  UseLastTableValue=on  InternalRulePriority=Speed  RndMeth=Simplest
  1-D Lookup Table1 : Lookup_n-D  NumberOfTableDimensions=1  BreakpointsForDimension1=longCTRparam.speed_vals_PID_sched  BeginIndexSearchUsingPreviousIndexResult=on  Table=longCTRparam.Ki_vals  ExtrapMethod=Clip  UseLastTableValue=on  InternalRulePriority=Speed  RndMeth=Simplest
  1-D Lookup Table2 : Lookup_n-D  NumberOfTableDimensions=1  BreakpointsForDimension1=longCTRparam.speed_vals_PID_sched  BeginIndexSearchUsingPreviousIndexResult=on  Table=longCTRparam.Kd_vals  ExtrapMethod=Clip  UseLastTableValue=on  InternalRulePriority=Speed  RndMeth=Simplest
  1-D Lookup Table3 : Lookup_n-D  NumberOfTableDimensions=1  BreakpointsForDimension1=longCTRparam.speed_vals_PID_sched  BeginIndexSearchUsingPreviousIndexResult=on  Table=longCTRparam.N_vals  ExtrapMethod=Clip  UseLastTableValue=on  InternalRulePriority=Speed  RndMeth=Simplest
  1-D Lookup Table4 : Lookup_n-D  NumberOfTableDimensions=1  BreakpointsForDimension1=longCTRparam.speed_vals_PID_sched  BeginIndexSearchUsingPreviousIndexResult=on  Table=longCTRparam.Kaw_vals  ExtrapMethod=Clip  UseLastTableValue=on  InternalRulePriority=Speed  RndMeth=Simplest
  Custom Low Level PID : Subsystem
  pedal_req : Outport  VectorParamsAs1DForOutWhenUnconnected=off
  wires:
  1-D Lookup Table/1 -> Custom Low Level PID/2(P)
  u_err/1 -> Custom Low Level PID/1(err)
  u_real/1 -> 1-D Lookup Table4/1, Custom Low Level PID/7(u_veh), 1-D Lookup Table3/1, 1-D Lookup Table2/1, 1-D Lookup Table1/1, 1-D Lookup Table/1
  1-D Lookup Table2/1 -> Custom Low Level PID/4(D)
  1-D Lookup Table3/1 -> Custom Low Level PID/5(N)
  1-D Lookup Table1/1 -> Custom Low Level PID/3(I)
  Custom Low Level PID/1(out_PID) -> pedal_req/1  "pedal_req"
  1-D Lookup Table4/1 -> Custom Low Level PID/6(Kaw)

== system Vehicle_Model_2Track_ABS_ESP_KINOBS_EMPTY/Estimate pose/Online Trajectory Plots ==
  targetPoint_steerCtrl : Inport
  pose : Inport  Port=2
  Enable : EnablePort
  Constant : Constant  Value=road_data_sampled
  Constant3 : Constant  Value=enable_zoom
  Constant5 : Constant  Value=latContr_select
  Plot manager : MATLAB Function  TreatAsAtomicUnit=on
  wires:
  targetPoint_steerCtrl/1 -> Plot manager/2(targetPoint_steerCtrl)
  Constant/1 -> Plot manager/4(refPath)
  Constant3/1 -> Plot manager/3(enable_zoomMPC)
  pose/1 -> Plot manager/1(vehiclePose)
  Constant5/1 -> Plot manager/5(latContr_type)

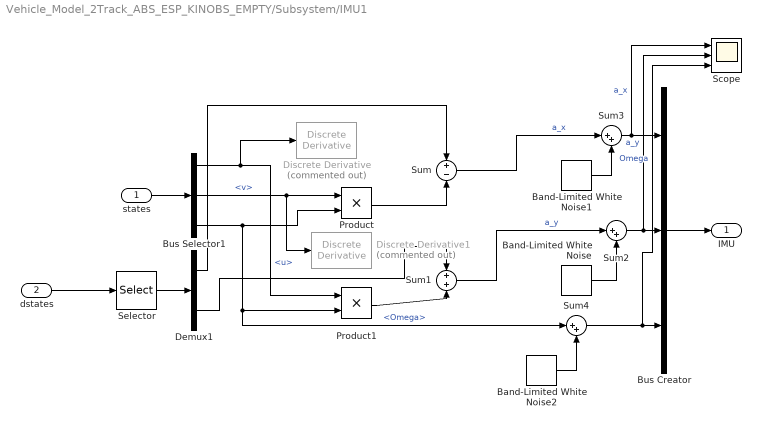
== system Vehicle_Model_2Track_ABS_ESP_KINOBS_EMPTY/Subsystem/IMU1 ==
  states : Inport
  dstates : Inport  Port=2
  Band-Limited White Noise : simulink/Sources/Band-Limited White Noise  Cov=[0.0001]  Ts=Ts  seed=[23341]
  Band-Limited White Noise1 : simulink/Sources/Band-Limited White Noise  Cov=[0.0001]  Ts=Ts  seed=[233241]
  Band-Limited White Noise2 : simulink/Sources/Band-Limited White Noise  Cov=[0.0001]  Ts=Ts  seed=[23341]
  Bus Creator : BusCreator  Inputs=3
  Bus Selector1 : BusSelector  OutputSignals=u,v,Omega
  Demux1 : Demux  Outputs=2
  Discrete Derivative : simulink/Discrete/Discrete Derivative  Commented=on  gainval=1.0  ICPrevScaledInput=0.0  OutMin=[]  OutMax=[]  OutDataType=fixdt(1, 16)  OutScaling=2^-10  DoSatur=off
  Discrete Derivative1 : simulink/Discrete/Discrete Derivative  Commented=on  gainval=1.0  ICPrevScaledInput=0.0  OutMin=[]  OutMax=[]  OutDataType=fixdt(1, 16)  OutScaling=2^-10  DoSatur=off
  Product : Product
  Product1 : Product
  Scope : Scope  NumInputPorts=3
  Selector : Selector  InputPortWidth=23  IndexOptions=Index vector (dialog)  Indices=[4 5]  OutputSizes=1
  Sum : Sum  Inputs=+-
  Sum1 : Sum
  Sum2 : Sum  Inputs=|++
  Sum3 : Sum  Inputs=|++
  Sum4 : Sum  Inputs=|++
  IMU : Outport
  wires:
  states/1 -> Bus Selector1/1
  Bus Selector1/1 -> Discrete Derivative/1, Product1/1  "<u>"
  Product/1 -> Sum/2
  Bus Selector1/2 -> Discrete Derivative1/1, Product/1  "<v>"
  Bus Selector1/3 -> Sum4/1, Product1/2, Product/2  "<Omega>"
  Sum/1 -> Sum3/1  "a_x"
  Product1/1 -> Sum1/2
  Sum1/1 -> Sum2/1  "a_y"
  Bus Creator/1 -> IMU/1
  dstates/1 -> Selector/1
  Selector/1 -> Demux1/1
  Demux1/2 -> Sum1/1
  Demux1/1 -> Sum/1
  Band-Limited White Noise/1 -> Sum2/2
  Sum2/1 -> Scope/2, Bus Creator/2  "a_y"
  Band-Limited White Noise1/1 -> Sum3/2
  Sum3/1 -> Scope/1, Bus Creator/1  "a_x"
  Sum4/1 -> Scope/3, Bus Creator/3  "Omega"
  Band-Limited White Noise2/1 -> Sum4/2

== system Vehicle_Model_2Track_ABS_ESP_KINOBS_EMPTY/Driver/Lateral Controller/Arc Path Following Controller ==
  targetPoint : Inport
  pose : Inport  Port=2
  endOfCircuit : Inport  Port=3
  Action Port : ActionPort  ActionPortLabel=case [ 1 ]:
  Arc Path Following Controller : MATLAB Function  TreatAsAtomicUnit=on
  delta : Outport  VectorParamsAs1DForOutWhenUnconnected=off
  wires:
  Arc Path Following Controller/1(delta) -> delta/1
  targetPoint/1 -> Arc Path Following Controller/1(target_Point)
  pose/1 -> Arc Path Following Controller/2(pose)
  endOfCircuit/1 -> Arc Path Following Controller/3(endOfCircuit)

== system Vehicle_Model_2Track_ABS_ESP_KINOBS_EMPTY/Driver/Lateral Controller/Lateral Controller Clothoid-based ==
  targetPoint : Inport
  pose : Inport  Port=2
  speed : Inport  Port=3
  endOfCircuit : Inport  Port=4
  Action Port : ActionPort  ActionPortLabel=case [ 4 ]:
  MATLAB System : MATLABSystem  System=clothoidBased_lateralController  lookAhead=clothoidBasedParams.lookAhead  Kus=clothoidBasedParams.Kus  L=vehicle_data.vehicle.L  SimulateUsing=Interpreted execution
      mask Type: clothoidBased_lateralController
      mask Display:
      | disp('clothoidBased_lateralController');
      | port_label('input',1,'targetPoint');
      | port_label('input',2,'vehPose');
      | port_label('input',3,'vehSpeed');
      | port_label('input',4,'endOfCircuit');
      | port_label('output',1,'delta_req');
  Selector : Selector  InputPortWidth=4  IndexOptions=Index vector (dialog)  Indices=[1 2 3]  OutputSizes=1
  delta : Outport  VectorParamsAs1DForOutWhenUnconnected=off
  wires:
  speed/1 -> MATLAB System/3
  MATLAB System/1 -> delta/1
  pose/1 -> MATLAB System/2
  targetPoint/1 -> Selector/1
  Selector/1 -> MATLAB System/1
  endOfCircuit/1 -> MATLAB System/4

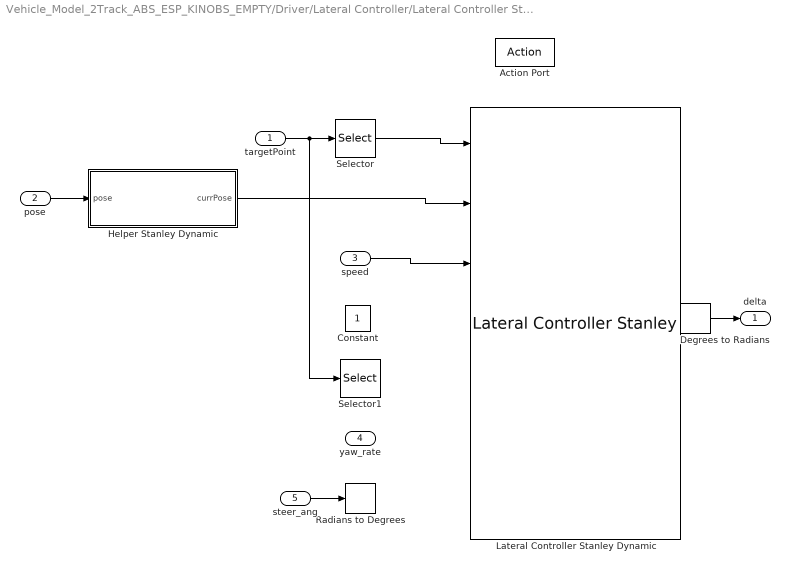
== system Vehicle_Model_2Track_ABS_ESP_KINOBS_EMPTY/Driver/Lateral Controller/Lateral Controller Stanley Dynamic ==
  targetPoint : Inport
  pose : Inport  Port=2
  speed : Inport  Port=3
  yaw_rate : Inport  Port=4
  steer_ang : Inport  Port=5
  Action Port : ActionPort  ActionPortLabel=case [ 3 ]:
  Constant : Constant
  Degrees to Radians : simulink_extras/Transformations/Degrees to Radians
  Helper Stanley Dynamic : MATLAB Function  TreatAsAtomicUnit=on
  Lateral Controller Stanley Dynamic : drivingvehiclecontroller/Lateral Controller Stanley  ModelType=Dynamic bicycle model  PositionGainF=stanleyParams.positGainFW  PositionGainR=stanleyParams.positGainREV  YawRateGain=stanleyParams.yawRateGain  DelayGain=stanleyParams.steerGain  VehicleMass=vehicle_data.vehicle.m  Lf=vehicle_data.vehicle.Lf  Lr=vehicle_data.vehicle.Lr  TireStiffness=stanleyParams.cornerStiff  Wheelbase=2.8  MaxSteeringAngle=stanleyParams.maxSteerAngle
  Radians to Degrees : simulink_extras/Transformations/Radians to Degrees
  Selector : Selector  InputPortWidth=4  IndexOptions=Index vector (dialog)  Indices=[1 2 3]  OutputSizes=1
  Selector1 : Selector  InputPortWidth=4  IndexOptions=Index vector (dialog)  Indices=[4]  OutputSizes=1
  delta : Outport  VectorParamsAs1DForOutWhenUnconnected=off
  wires:
  Lateral Controller Stanley Dynamic/1 -> Degrees to Radians/1
  pose/1 -> Helper Stanley Dynamic/1(pose)
  speed/1 -> Lateral Controller Stanley Dynamic/3
  Degrees to Radians/1 -> delta/1
  Helper Stanley Dynamic/1(currPose) -> Lateral Controller Stanley Dynamic/2
  targetPoint/1 -> Selector1/1, Selector/1
  Selector/1 -> Lateral Controller Stanley Dynamic/1
  steer_ang/1 -> Radians to Degrees/1

== system Vehicle_Model_2Track_ABS_ESP_KINOBS_EMPTY/Driver/Lateral Controller/Lateral Controller Stanley Kinematic ==
  targetPoint : Inport
  pose : Inport  Port=2
  speed : Inport  Port=3
  Action Port : ActionPort  ActionPortLabel=case [ 2 ]:
  Constant : Constant
  Degrees to Radians : simulink_extras/Transformations/Degrees to Radians
  Helper Stanley Kinematic : MATLAB Function  TreatAsAtomicUnit=on
  Lateral Controller Stanley Kinematic : drivingvehiclecontroller/Lateral Controller Stanley  ModelType=Kinematic bicycle model  PositionGainF=stanleyParams.positGainFW  PositionGainR=stanleyParams.positGainREV  YawRateGain=0.2  DelayGain=0.2  VehicleMass=1575  Lf=1.2  Lr=1.6  TireStiffness=19000  Wheelbase=vehicle_data.vehicle.Lf + vehicle_data.vehicle.Lr  MaxSteeringAngle=stanleyParams.maxSteerAngle
  Selector : Selector  InputPortWidth=4  IndexOptions=Index vector (dialog)  Indices=[1 2 3]  OutputSizes=1
  delta : Outport  VectorParamsAs1DForOutWhenUnconnected=off
  wires:
  Lateral Controller Stanley Kinematic/1 -> Degrees to Radians/1
  pose/1 -> Helper Stanley Kinematic/1(pose)
  speed/1 -> Lateral Controller Stanley Kinematic/3
  Constant/1 -> Lateral Controller Stanley Kinematic/4
  Degrees to Radians/1 -> delta/1
  Helper Stanley Kinematic/1(currPose) -> Lateral Controller Stanley Kinematic/2
  targetPoint/1 -> Selector/1
  Selector/1 -> Lateral Controller Stanley Kinematic/1

== system Vehicle_Model_2Track_ABS_ESP_KINOBS_EMPTY/Driver/Lateral Controller/Preview point lateral Controller ==
  targetPoint : Inport
  endOfCircuit : Inport  Port=2
  Action Port : ActionPort  ActionPortLabel=case [ 5 ]:
  Constant : Constant  Value=previewPointParams.ke
  Constant1 : Constant  Value=previewPointParams.kp
  Preview Point Controller : MATLAB Function  TreatAsAtomicUnit=on
  delta : Outport  VectorParamsAs1DForOutWhenUnconnected=off
  wires:
  Preview Point Controller/1(delta) -> delta/1
  targetPoint/1 -> Preview Point Controller/1(target_Point)
  endOfCircuit/1 -> Preview Point Controller/4(endOfCircuit)
  Constant/1 -> Preview Point Controller/2(ke)
  Constant1/1 -> Preview Point Controller/3(kp)

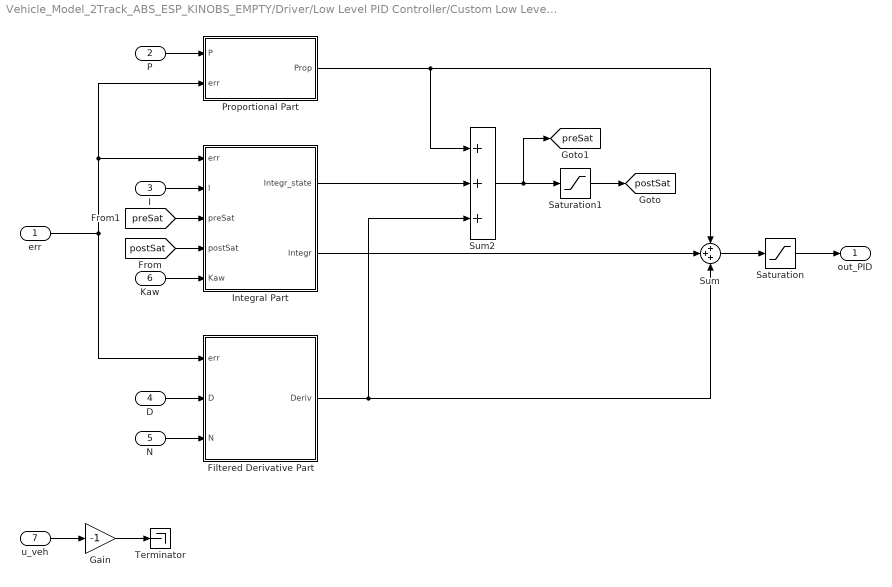
== system Vehicle_Model_2Track_ABS_ESP_KINOBS_EMPTY/Driver/Low Level PID Controller/Custom Low Level PID ==
  err : Inport
  P : Inport  Port=2
  I : Inport  Port=3
  D : Inport  Port=4
  N : Inport  Port=5
  Kaw : Inport  Port=6
  u_veh : Inport  Port=7
  Filtered Derivative Part : Subsystem
  Gain : Gain  Gain=-1
  Integral Part : Subsystem
  Proportional Part : Subsystem
  Saturation : Saturate  UpperLimit=1  LowerLimit=-1  LinearizeAsGain=off
  Saturation1 : Saturate  UpperLimit=1  LowerLimit=-1  LinearizeAsGain=off
  Sum : Sum  Inputs=+++
  Sum2 : Sum  Inputs=+++
  Terminator : Terminator
  out_PID : Outport  VectorParamsAs1DForOutWhenUnconnected=off
  tag scope: postSat=global, preSat=global
  wires:
  Sum2/1 -> [preSat], Saturation1/1
  Sum/1 -> Saturation/1
  Saturation/1 -> out_PID/1
  err/1 -> Filtered Derivative Part/1(err), Proportional Part/2(err), Integral Part/1(err)
  Saturation1/1 -> [postSat]
  I/1 -> Integral Part/2(I)
  Integral Part/1(Integr_state) -> Sum2/2
  Integral Part/2(Integr) -> Sum/2
  Proportional Part/1(Prop) -> Sum2/1, Sum/1
  P/1 -> Proportional Part/1(P)
  [preSat] -> Integral Part/3(preSat)
  [postSat] -> Integral Part/4(postSat)
  Filtered Derivative Part/1(Deriv) -> Sum/3, Sum2/3
  D/1 -> Filtered Derivative Part/2(D)
  N/1 -> Filtered Derivative Part/3(N)
  u_veh/1 -> Gain/1
  Gain/1 -> Terminator/1
  Kaw/1 -> Integral Part/5(Kaw)

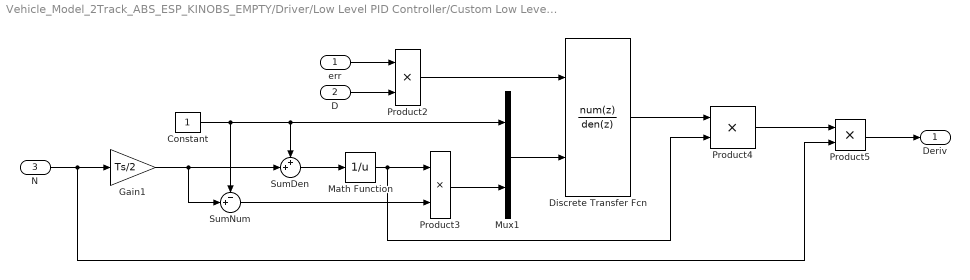
== system Vehicle_Model_2Track_ABS_ESP_KINOBS_EMPTY/Driver/Low Level PID Controller/Custom Low Level PID/Filtered Derivative Part ==
  err : Inport
  D : Inport  Port=2
  N : Inport  Port=3
  Constant : Constant
  Discrete Transfer Fcn : DiscreteTransferFcn  Numerator=[1 -1]  DenominatorSource=Input port  SampleTime=Ts  a0EqualsOne=on
      settings: InputPortMap=u0,p3
  Gain1 : Gain  Gain=Ts/2
  Math Function : Math  Operator=reciprocal  SignedPower=on
  Mux1 : Mux  Inputs=2
  Product{2..5} (4 alike) : Product
  SumDen : Sum  Inputs=++|
  SumNum : Sum  Inputs=-+|
  Deriv : Outport  VectorParamsAs1DForOutWhenUnconnected=off
  wires:
  N/1 -> Gain1/1, Product5/2
  Product4/1 -> Product5/1
  SumDen/1 -> Math Function/1
  Math Function/1 -> Product4/2, Product3/1
  SumNum/1 -> Product3/2
  Product2/1 -> Discrete Transfer Fcn/1
  Discrete Transfer Fcn/1 -> Product4/1
  Constant/1 -> SumNum/1, SumDen/1, Mux1/1
  Product3/1 -> Mux1/2
  Mux1/1 -> Discrete Transfer Fcn/2
  Gain1/1 -> SumNum/2, SumDen/2
  err/1 -> Product2/1
  D/1 -> Product2/2
  Product5/1 -> Deriv/1

== system Vehicle_Model_2Track_ABS_ESP_KINOBS_EMPTY/Driver/Low Level PID Controller/Custom Low Level PID/Integral Part ==
  err : Inport
  I : Inport  Port=2
  preSat : Inport  Port=3
  postSat : Inport  Port=4
  Kaw : Inport  Port=5
  Anti-windup : Subsystem
  Discrete-Time Integrator1 : DiscreteIntegrator  IntegratorMethod=Integration: Trapezoidal  SampleTime=Ts  ShowStatePort=on  ICPrevOutput=DiscIntNeverNeededParam  ICPrevScaledInput=DiscIntNeverNeededParam
  Product1 : Product
  Integr_state : Outport  VectorParamsAs1DForOutWhenUnconnected=off
  Integr : Outport  Port=2  VectorParamsAs1DForOutWhenUnconnected=off
  wires:
  Discrete-Time Integrator1/State -> Integr_state/1
  preSat/1 -> Anti-windup/2(preSat)
  Product1/1 -> Anti-windup/4(preInt)
  postSat/1 -> Anti-windup/3(postSat)
  I/1 -> Product1/2
  Anti-windup/1(Out_antiWindUp) -> Discrete-Time Integrator1/1
  Discrete-Time Integrator1/1 -> Integr/1
  err/1 -> Product1/1
  Kaw/1 -> Anti-windup/1(Kaw)

== system Vehicle_Model_2Track_ABS_ESP_KINOBS_EMPTY/Driver/Low Level PID Controller/Custom Low Level PID/Proportional Part ==
  P : Inport
  err : Inport  Port=2
  Product : Product
  Prop : Outport  VectorParamsAs1DForOutWhenUnconnected=off
  wires:
  P/1 -> Product/2
  Product/1 -> Prop/1
  err/1 -> Product/1

== system Vehicle_Model_2Track_ABS_ESP_KINOBS_EMPTY/Driver/Low Level PID Controller/Custom Low Level PID/Integral Part/Anti-windup ==
  Kaw : Inport
  preSat : Inport  Port=2
  postSat : Inport  Port=3
  preInt : Inport  Port=4
  Product : Product
  Sum : Sum  Inputs=|-+
  Sum1 : Sum  Inputs=|++
  Out_antiWindUp : Outport  VectorParamsAs1DForOutWhenUnconnected=off
  wires:
  preSat/1 -> Sum/1
  preInt/1 -> Sum1/2
  Product/1 -> Sum1/1
  Sum1/1 -> Out_antiWindUp/1
  Sum/1 -> Product/2
  postSat/1 -> Sum/2
  Kaw/1 -> Product/1

== matlab function Vehicle_Model_2Track_ABS_ESP_KINOBS_EMPTY/ABS and Wheel torque generation/ESP/dmax ==
  data: u input; beta_dmax output; mu input; gamma_dmax output; X input; extra_params input; vehicle_data parameter
function [beta_dmax, gamma_dmax] = dmax(u, mu, X, extra_params, vehicle_data)

  Lf = vehicle_data.vehicle.Lf;  % [m] Distance between vehicle CoG and front wheels axle
    Lr = vehicle_data.vehicle.Lr;  % [m] Distance between vehicle CoG and front wheels axle
    L  = vehicle_data.vehicle.L;   % [m] Vehicle length
    Wf = vehicle_data.vehicle.Wf;  % [m] Width of front wheels axle 
    Wr = vehicle_data.vehicle.Wr;  % [m] Width of rear wheels axle                   
    m  = vehicle_data.vehicle.m;   % [kg] Vehicle Mass
    g  = vehicle_data.vehicle.g;   % [m/s^2] Gravitational acceleration
    hs = vehicle_data.vehicle.hGs;
    izz= vehicle_data.vehicle.i_zz;

v         = X(5);       % [m/s] vehicle lateral speed
gamma     = X(6);       % [rad/s] yaw rate
Fz__rr    = X(7);       % [N] vertical force for the rear right wheel
Fz__rl    = X(8);       % [N] vertical force for the rear left wheel
Fz__fr    = X(9);       % [N] vertical force for the front right wheel
Fz__fl    = X(10);      % [N] vertical force for the front left wheel
delta     = X(11);      % [rad] steering angle (at the wheel)

  

alpha__rr = X(16);      % [rad] side slip angle rear right wheel
alpha__rl = X(17);      % [rad] side slip angle rear left wheel
alpha__fr = X(18);      % [rad] side slip angle front right wheel
alpha__fl = X(19);      % [rad] side slip angle front left wheel

    
Fy__rr = extra_params(9);
Fy__rl = extra_params(10);
Fy__fr = extra_params(11);
Fy__fl = extra_params(12);

% if(alpha__rr < 10^-3 && alpha__fr < 10^-3)
%     alpha__fr = 3*10^-1;
%     alpha__rr = 10^-1;
% end

C_fl = (Fy__fl)./(alpha__fl);
C_fr = (Fy__fr)./(alpha__fr);
C_rl = (Fy__rl)./(alpha__rl);
C_rr = (Fy__rr)./(alpha__rr);

C_f = C_fl + C_fr;
C_r = C_rl + C_rr;

gamma_dmax = mu.*g./u;
beta_dmax = mu.*g.*(Lr./u.^2 + m.*Lf./(C_r.*L));

== matlab function Vehicle_Model_2Track_ABS_ESP_KINOBS_EMPTY/ABS and Wheel torque generation/ESP/ASC ==
  data: delta input; X input; extra_params input; beta_ref input; gamma_ref input; Mz output; vehicle_data parameter
function Mz = asc(delta, X, extra_params, beta_ref, gamma_ref, vehicle_data)

 Lf = vehicle_data.vehicle.Lf;  % [m] Distance between vehicle CoG and front wheels axle
    Lr = vehicle_data.vehicle.Lr;  % [m] Distance between vehicle CoG and front wheels axle
    L  = vehicle_data.vehicle.L;   % [m] Vehicle length
    Wf = vehicle_data.vehicle.Wf;  % [m] Width of front wheels axle 
    Wr = vehicle_data.vehicle.Wr;  % [m] Width of rear wheels axle                   
    m  = vehicle_data.vehicle.m;   % [kg] Vehicle Mass
    g  = vehicle_data.vehicle.g;   % [m/s^2] Gravitational acceleration
    hs = vehicle_data.vehicle.hGs;
    izz= vehicle_data.vehicle.i_zz;

u         = X(4);       % [m/s] vehicle longitudinal speed
v         = X(5);       % [m/s] vehicle lateral speed
gamma     = X(6);       % [rad/s] yaw rate

Fx__fr = extra_params(7);
Fx__fl = extra_params(8);

beta = atan2(v, u);
beta_dot = 0.0;

gamma_dot_ref = 1e-4;
beta_dot_ref = 1e-4;

xi = 0.2;
S = gamma - gamma_ref + xi.*(beta - beta_ref);

k_p = 8.0;
k_s = 0.5;

Mz = -Lf.*(Fx__fr + Fx__fl).*sin(delta) - izz.*(k_p.*S + k_s.*sign(S) - gamma_dot_ref + xi.*(beta_dot - beta_dot_ref));

== matlab function Vehicle_Model_2Track_ABS_ESP_KINOBS_EMPTY/ABS and Wheel torque generation/ESP/Torque ==
  data: Mz input; T1 output; X input; dX input; T2 output; T3 output; T4 output; vehicle_data parameter; Tq output
function [T1, T2, T3, T4, Tq] = consmin(Mz, X, dX, vehicle_data)

Wf = vehicle_data.vehicle.Wf;  % [m] Width of front wheels axle 
Wr = vehicle_data.vehicle.Wr;  % [m] Width of rear wheels axle                   
m  = vehicle_data.vehicle.m;   % [kg] Vehicle Mass
g  = vehicle_data.vehicle.g;   % [m/s^2] Gravitational acceleration

Fz__rr    = X(7);       % [N] vertical force for the rear right wheel
Fz__rl    = X(8);       % [N] vertical force for the rear left wheel
Fz__fr    = X(9);       % [N] vertical force for the front right wheel
Fz__fl    = X(10);      % [N] vertical force for the front left wheel

R = 0.3270;
u_dot = dX(4);
Tq = m.*u_dot./R;
mu = 0.8;

B = [ 1,  1,  1,  1;
    -Wf/(2.*R),  Wf/(2.*R),  -Wr/(2.*R),  Wr/(2.*R) ];
% B = [];

% if(Mz < 10^-3)
%     Mz = 10;
% end

% if(Tq < 10^-3)
%     Tq = 10;
% end

if(Mz > 10^7)
    Mz = 10^4;
end

if(Tq > 10^7)
    Tq = 10^3;
end

Mz(isinf(Mz)|isnan(Mz)) = 10^3;

v_c = [Tq; Mz];
% v_c = [10;10];

lb = [-mu.*Fz__fl.*R, -mu.*Fz__fr.*R ,-mu.*Fz__rl.*R, -mu.*Fz__rr.*R];

ub = [mu.*Fz__fl.*R, mu.*Fz__fr.*R, mu.*Fz__rl.*R, mu.*Fz__rr.*R];

options = optimoptions('fmincon','Display','iter','Algorithm','sqp');

fun = @(T)T(1).^2./(mu.*Fz__fl.*R).^2 + T(2).^2./(mu.*Fz__fr.*R).^2 + T(3).^2./(mu.*Fz__rl.*R).^2 + T(4).^2./(mu.*Fz__rr.*R).^2;

T = fmincon(fun, [1, 1, 1, 1], [], [], B, v_c, lb, ub , [], options);

T1 = T(1);
T2 = T(2);
T3 = T(3);
T4 = T(4);

% T1 = 0;
% T2 = 0;
% T3 = 0;
% T4 = 0;
